simulink model "Droop"  (R2024b)
settings: Solver=VariableStepAuto  StartTime=0.0  StopTime=2  RelTol=1e-3
undefined symbols (not defined in the file): Ion, Lithium
libraries: spsSeriesRLCBranchLib x7, spsVoltageMeasurementLib x6, spsMosfetLib x4, spsCurrentMeasurementLib x3, spsBatteryLib x2, slpidlib x2, spsTriangleGeneratorLib x2, spsBreakerLib x1, spsPVArrayLib x1, spspowerguiLib x1
settings Model: Creator=ASUS  LastModifiedBy=ASUS

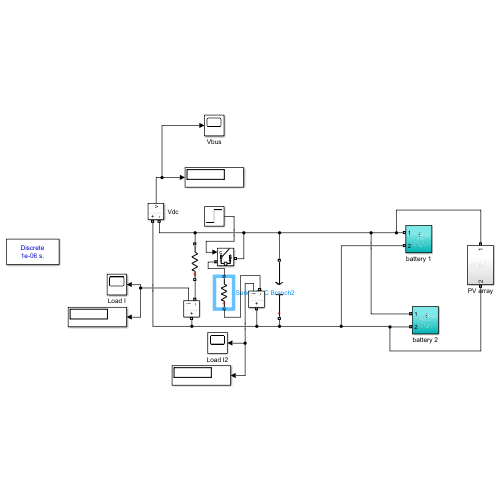
[thumbnail: Simulink's stored preview of the top-level diagram]
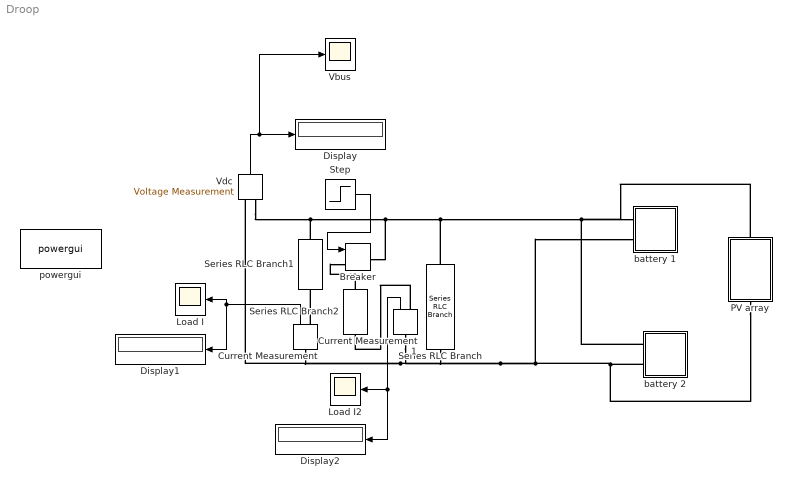
== system Droop ==
  Breaker : spsBreakerLib/Breaker  InitialState=0  SwitchingTimes="[1/60  5/60]"  External=on  BreakerResistance=0.01  SnubberResistance=1e6  SnubberCapacitance=inf  Measurements=None  MoreParameters=on  NoBreakLoop=off
  Current Measurement : spsCurrentMeasurementLib/Current Measurement  PhasorSimulation=off  OutputType=Complex  PSBequivalent=0
  Current Measurement1 : spsCurrentMeasurementLib/Current Measurement  PhasorSimulation=off  OutputType=Complex  PSBequivalent=0
  Display : Display
  Display1 : Display
  Display2 : Display
  Load I : Scope
  Load I2 : Scope
  PV array : Subsystem
      settings: PortSchema="{\"entries\":[{\"content\":{\"sides\":[{\"content\":{},\"type\":\"ConnectorPlacement.EquallySpacedRectSide\",\"uuid\":\"98c84815-b73a-4a68-a881-ea3acd4700a6\"},{\"content\":{\"side\":\"RIGHT\"},\"type\":\"ConnectorPlacement.EquallySpacedRectSide\",\"uuid\":\"a3c80d2d-1955-4a58-b743-6cecb5515e4f\"},{\"content\":{\"connectorIds\":[\"LConn1\"],\"side\":\"TOP\"},\"type\":\"ConnectorPlacement.EquallySpacedRectSide\",\"uuid\":\"fb99ad30-251c-48f2-b563-c26654c12262\"},{\"content\":{\"connectorIds\":[\"RConn1\"],\"side\":\"BOTTOM\"},\"type\":\"ConnectorPlacement.EquallySpacedRectSide\",\"uuid\":\"3c114dca-ead0-42e1-8f9f-90199643fe12\"}]},\"type\":\"ConnectorPlacement.EquallySpacedConnector\",\"uuid\":\"efc59635-4512-4ae2-8e03-d54fb94518f3\"}],\"packageUris\":[\"http://schema.mathworks.com/mf0/Connector/R2020b\"],\"version\":\"1.0\"}"
  Series RLC Branch : spsSeriesRLCBranchLib/Series RLC Branch  LConnTagsString=__new0  RConnTagsString=__new0  BranchType=C  Resistance=1  Inductance=1e-3  SetiL0=off  InitialCurrent=0  Capacitance=4700e-6  Setx0=off  InitialVoltage=0  Measurements=None
  Series RLC Branch1 : spsSeriesRLCBranchLib/Series RLC Branch  LConnTagsString=__new0  RConnTagsString=__new0  BranchType=R  Resistance=1  Inductance=1e-3  SetiL0=off  InitialCurrent=0  Capacitance=4700e-6  Setx0=off  InitialVoltage=0  Measurements=None
  Series RLC Branch2 : spsSeriesRLCBranchLib/Series RLC Branch  LConnTagsString=__new0  RConnTagsString=__new0  BranchType=R  Resistance=1  Inductance=1e-3  SetiL0=off  InitialCurrent=0  Capacitance=4700e-6  Setx0=off  InitialVoltage=0  Measurements=None
  Step : Step  Time=0.5  SampleTime=0
  Vbus : Scope
  Vdc : spsVoltageMeasurementLib/Voltage Measurement  PhasorSimulation=off  OutputType=Complex  PSBequivalent=0
  battery 1 : Subsystem
  battery 2 : Subsystem
  powergui : spspowerguiLib/powergui  Priority=1  SimulationMode=Discrete  SampleTime=1e-6  frequency=60  Iterations=50  frequencyindice=0  Pbase=100e6  ErrMax=1e-4  UnitsV=kV  UnitsW=MW  buscounter=0  FunctionMessages=off  echomessages=off  EnableUseOfTLC=off  CurrentSourceSwitches=off  DisableSnubberDevices=off  DisableRonSwitches=off  DisableVfSwitches=off  DisplayEquations=off  AutomaticDiscreteSolvers=off  SolverType=Tustin/Backward Euler (TBE)  Interpol=off  ExternalGateDelay=off  methode=off  Ts=100  x0status=blocks  SPID=on  SwTol=0  HookPort=off  NonlinearTolerance=1e-4  nMaxIteration=100  ContinueOnMaxIteration=off  RestoreLinks=warning  ResistiveCurrentMeasurement=off  Frange=[0:2:500]  Ylog=off  Xlog=on  ShowGrid=off  save=off  variable=ZData  structure=0  ZoomFFT=off  StartTime=0.0  cycles=1  DisplayStyle=1  fundamental=60  FreqAxis=off  MaxFrequency=1000  frequencyindicesteady=1  RmsSteady=1  display=off
  wires:
  Vdc/1 -> Vbus/1, Display/1
  Step/1 -> Breaker/1
  Current Measurement/1 -> Load I/1, Display1/1
  Current Measurement1/1 -> Display2/1, Load I2/1
  connections:
  battery 2/LConn2 -- battery 1/LConn2 -- Current Measurement/LConn1 -- Vdc/LConn1 -- Current Measurement1/LConn1 -- Series RLC Branch/LConn1 -- PV array/RConn1
  Vdc/LConn2 -- Series RLC Branch1/RConn1 -- Breaker/RConn1 -- Series RLC Branch/RConn1 -- PV array/LConn1 -- battery 1/LConn1 -- battery 2/LConn1
  Series RLC Branch2/RConn1 -- Breaker/LConn1
  Current Measurement/RConn1 -- Series RLC Branch1/LConn1
  Current Measurement1/RConn1 -- Series RLC Branch2/LConn1

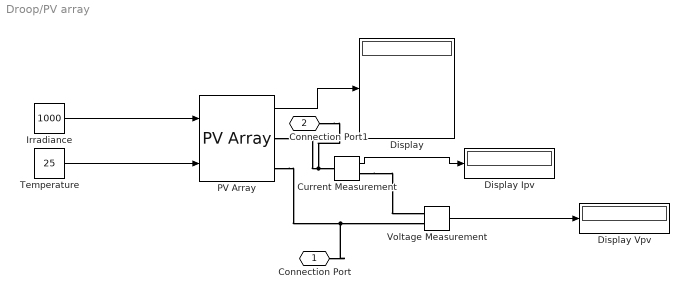
== system Droop/PV array ==
  Current Measurement : spsCurrentMeasurementLib/Current Measurement  PhasorSimulation=off  OutputType=Complex  PSBequivalent=0
  Display : Display
  Display Ipv : Display
  Display Vpv : Display
  Irradiance : Constant  Value=1000
  PV Array : spsPVArrayLib/PV Array  Npar=40  Nser=10  PlotType=array @ 1000 W/m2 & specified temperatures  S_vec="[ 1000  500  100 ]"  Temp_C_vec="[ 45 25  ]"  ModuleName=SunPower SPR-295E-WHT-D  PlotWhenSelected=off  Pm=295.39  Ncell=96  Voc=63.3  Isc=5.83  Vm=54.2  Im=5.45  beta_Voc_pc=-0.2727  alpha_Isc_pc=0.061732  beta_Voc=-0.17262  alpha_Isc=0.003599  IL=5.8532  I0=6.1666e-12  nI=0.93176  Rsh=315.2663  Rs=0.32243  RobustModel=off  RobustCellTemperature=313.3991  BAL=off  Tc=1e-6  Tfilter=5e-5
  Temperature : Constant  Value=25
  Voltage Measurement : spsVoltageMeasurementLib/Voltage Measurement  PhasorSimulation=off  OutputType=Complex  PSBequivalent=0
  Connection Port : PMIOPort  Side=Left
  Connection Port1 : PMIOPort  Port=2  Side=Right
  wires:
  Temperature/1 -> PV Array/2
  PV Array/1 -> Display/1
  Voltage Measurement/1 -> Display Vpv/1
  Irradiance/1 -> PV Array/1
  Current Measurement/1 -> Display Ipv/1
  connections:
  Current Measurement/RConn1 -- Voltage Measurement/LConn1
  PV Array/RConn2 -- Connection Port/RConn1 -- Voltage Measurement/LConn2
  PV Array/RConn1 -- Connection Port1/RConn1 -- Current Measurement/LConn1

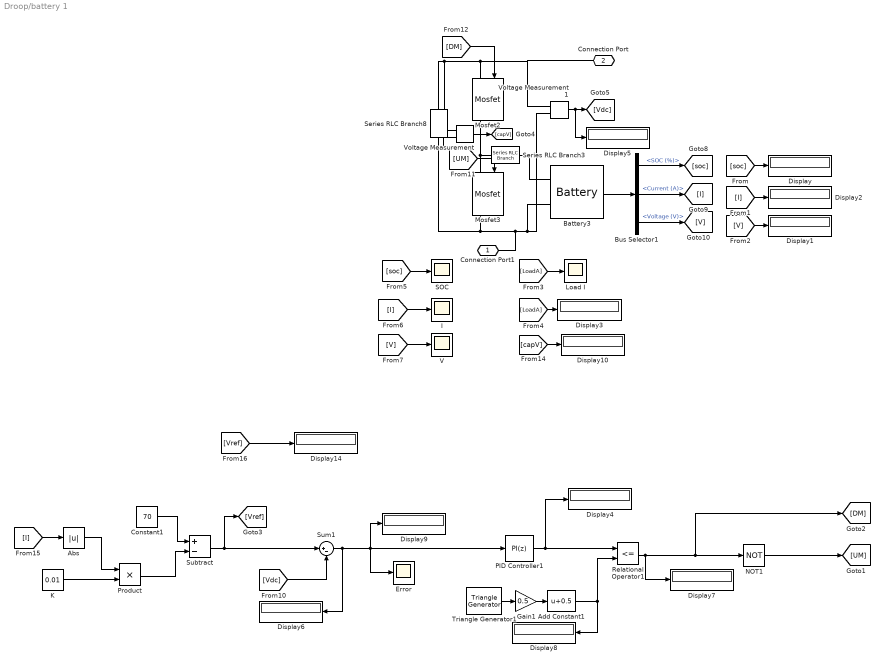
== system Droop/battery 1 ==
  Abs : Abs  SaturateOnIntegerOverflow=off
  Add Constant1 : Bias  Bias=0.5  SaturateOnIntegerOverflow=off
  Battery3 : spsBatteryLib/Battery  BatType=Lithium-Ion  NomV=50  NomQ=20  SOC=60  Batt_Tr=30  PresetModel=on  MaxQ=20  MinV=37.5  FullV=58.1994  Dis_rate=8.6957  R=0.025  Normal_OP=18.087  expZone="[54.0193     0.982609]"
  Bus Selector1 : BusSelector  OutputSignals=SOC (%),Current (A),Voltage (V)
  Constant1 : Constant  Value=70
  Display{,1..10,14} (12 alike) : Display
  Error : Scope
  Gain1 : Gain  Gain=0.5
  I : Scope
  K : Constant  Value=0.01
  Load I : Scope
  Mosfet2 : spsMosfetLib/Mosfet  Ron=0.1  Lon=0  Rd=0.01  Vfd=0  IC=0  Rs=1e6  Cs=inf  Measurements=on
  Mosfet3 : spsMosfetLib/Mosfet  Ron=0.1  Lon=0  Rd=0.01  Vfd=0  IC=0  Rs=1e6  Cs=inf  Measurements=on
  NOT1 : Logic  Operator=NOT  IconShape=distinctive  AllPortsSameDT=off  OutDataTypeStr=boolean
  PID Controller1 : slpidlib/PID Controller  Controller=PI  Form=Parallel  TimeDomain=Discrete-time  UseExternalTs=off  SampleTime=-1  IntegratorMethod=Forward Euler  FilterMethod=Forward Euler  ControllerParametersSource=internal  P=0.08  I=10  UseKiTs=off  D=0  UseExternalDerivativeSource=off  N=100  UseFilter=on  TunerSelectOption=Transfer Function Based (PID Tuner App)  ZeroCross=off  InitialConditionSource=internal  InitialConditionForIntegrator=0  InitialConditionForFilter=0  DifferentiatorICPrevScaledInput=0  ExternalReset=none  TrackingMode=off  Kt=1  LimitOutput=on  SatLimitsSource=internal  UpperSaturationLimit=1  LowerSaturationLimit=-1  LinearizeAsGain=on  AntiWindupMode=back-calculation  Kb=1  LimitIntegrator=off  UpperIntegratorSaturationLimit=inf  LowerIntegratorSaturationLimit=-inf  POutMin=[]  POutMax=[]  IOutMin=[]  IOutMax=[]  DOutMin=[]  DOutMax=[]  NOutMin=[]  NOutMax=[]  SumOutMin=[]  SumOutMax=[]  SaturationOutMin=[]  SaturationOutMax=[]  PParamMin=[]  PParamMax=[]  IParamMin=[]  IParamMax=[]  DParamMin=[]  DParamMax=[]  NParamMin=[]  NParamMax=[]  KbParamMin=[]  KbParamMax=[]  KtParamMin=[]  KtParamMax=[]  KbOutMin=[]  KbOutMax=[]  KtOutMin=[]  KtOutMax=[]  IntegratorOutMin=[]  IntegratorOutMax=[]  FilterOutMin=[]  FilterOutMax=[]  SumI1OutMin=[]  SumI1OutMax=[]  SumI2OutMin=[]  SumI2OutMax=[]  SumI3OutMin=[]  SumI3OutMax=[]  SumI4OutMin=[]  SumI4OutMax=[]  SumDOutMin=[]  SumDOutMax=[]  DifferentiatorOutMin=[]  DifferentiatorOutMax=[]  FilterDiffOutCoefMin=[]  FilterDiffOutCoefMax=[]  ReciprocalOutMin=[]  ReciprocalOutMax=[]  SumDenOutMin=[]  SumDenOutMax=[]  SumNumOutMin=[]  SumNumOutMax=[]  DivideOutMin=[]  DivideOutMax=[]  UdiffTsProdOutMin=[]  UdiffTsProdOutMax=[]  NTsProdOutMin=[]  NTsProdOutMax=[]  UintegralTsProdOutMin=[]  UintegralTsProdOutMax=[]  UngainTsProdOutMin=[]  UngainTsProdOutMax=[]  ClampingZeroOutDataTypeStr=Inherit: Inherit via back propagation  ClampingZeroOutMin=[]  ClampingZeroOutMax=[]  FilterDenConstantOutDataTypeStr=Inherit: Inherit via back propagation  FilterDenConstantOutMin=[]  FilterDenConstantOutMax=[]  PCopyOutDataTypeStr=Inherit: Inherit via back propagation  PCopyOutMin=[]  PCopyOutMax=[]  NCopyOutDataTypeStr=Inherit: Inherit via back propagation  NCopyOutMin=[]  NCopyOutMax=[]  IntegratorContinuousStateAttributes=''  IntegratorStateMustResolveToSignalObject=off  IntegratorRTWStateStorageClass=Auto  FilterContinuousStateAttributes=''  FilterStateMustResolveToSignalObject=off  FilterRTWStateStorageClass=Auto  ParallelPVariant=InternalParameters  IdealPVariant=Disabled  IVariant=InternalParameters  DVariant=Disabled  IntegratorVariant=Discrete  SatVariant=Enabled  AWVariant=BackCalculation  PCopyVariant=Disabled  TRVariant=Disabled  FdbkBlocksVariant=Forward  IdealPFdbkVariant=Disabled  SatFdbkVariant=Disabled  DerivativeFilterVariant=Disabled  NVariant=Disabled  NCopyVariant=Disabled_SignalSpec  FilterICVariant=Disabled  IntegratorICVariant=InternalICs  ExternalResetVariant=Disabled  TRSumVariant=Passthrough  SumFdbkVariant=Disabled  SumVariant=Sum_PI  TsampFilterVariant=InternalTs  TsampNgainVariant=Passthrough  TsampIntegralVariant=Disabled_SignalSpec  ExternalSaturationOutDataTypeStr=Inherit: Same as second input  DerivativeSourceVariant=Disabled  PreIntVariant=InternalPreInt
  Product : Product
  Relational Operator1 : RelationalOperator  Operator=<=  OutDataTypeStr=boolean  RndMeth=Simplest  InputSameDT=off
  SOC : Scope
  Series RLC Branch3 : spsSeriesRLCBranchLib/Series RLC Branch  LConnTagsString=__new0  RConnTagsString=__new0  BranchType=L  Resistance=1  Inductance=500e-6  SetiL0=off  InitialCurrent=0  Capacitance=1e-6  Setx0=off  InitialVoltage=0  Measurements=None
  Series RLC Branch8 : spsSeriesRLCBranchLib/Series RLC Branch  LConnTagsString=__new0  RConnTagsString=__new0  BranchType=RC  Resistance=1  Inductance=1e-3  SetiL0=off  InitialCurrent=0  Capacitance=1500e-6  Setx0=off  InitialVoltage=0  Measurements=None
  Subtract : Sum  Inputs=+-
  Sum1 : Sum  Inputs=|+-
  Triangle Generator1 : spsTriangleGeneratorLib/Triangle Generator  Freq=10000  Phase=0  Ts=1e-6
  V : Scope
  Voltage Measurement : spsVoltageMeasurementLib/Voltage Measurement  PhasorSimulation=off  OutputType=Complex  PSBequivalent=0
  Voltage Measurement1 : spsVoltageMeasurementLib/Voltage Measurement  PhasorSimulation=off  OutputType=Complex  PSBequivalent=0
  Connection Port1 : PMIOPort  Side=Left
  Connection Port : PMIOPort  Port=2  Side=Left
  wires:
  Voltage Measurement1/1 -> Display5/1, [Vdc]
  [UM] -> Mosfet3/1
  Add Constant1/1 -> Display8/1, Relational Operator1/2
  [V] -> Display1/1
  [capV] -> Display10/1
  [I] -> I/1
  Sum1/1 -> Display9/1, PID Controller1/1, Error/1, Display6/1
  Relational Operator1/1 -> [DM], NOT1/1, Display7/1
  Bus Selector1/1 -> [soc]  "<SOC (%)>"
  PID Controller1/1 -> Relational Operator1/1, Display4/1
  Gain1/1 -> Add Constant1/1
  [soc] -> SOC/1
  [I] -> Display2/1
  Battery3/1 -> Bus Selector1/1
  [DM] -> Mosfet2/1
  Bus Selector1/3 -> [V]  "<Voltage (V)>"
  [LoadA] -> Load I/1
  [V] -> V/1
  Voltage Measurement/1 -> [capV]
  [Vdc] -> Sum1/2
  [LoadA] -> Display3/1
  Triangle Generator1/1 -> Gain1/1
  Subtract/1 -> Sum1/1, [Vref]
  Bus Selector1/2 -> [I]  "<Current (A)>"
  [soc] -> Display/1
  [I] -> Abs/1
  Abs/1 -> Product/1
  K/1 -> Product/2
  Product/1 -> Subtract/2
  Constant1/1 -> Subtract/1
  NOT1/1 -> [UM]
  [Vref] -> Display14/1
  connections:
  Battery3/LConn1 -- Series RLC Branch3/LConn1
  Series RLC Branch8/LConn1 -- Voltage Measurement1/LConn1 -- Connection Port/RConn1 -- Mosfet2/LConn1 -- Voltage Measurement/LConn1
  Battery3/LConn2 -- Connection Port1/RConn1 -- Series RLC Branch8/RConn1 -- Voltage Measurement/LConn2 -- Mosfet3/RConn1 -- Voltage Measurement1/LConn2
  Mosfet2/RConn1 -- Series RLC Branch3/RConn1 -- Mosfet3/LConn1

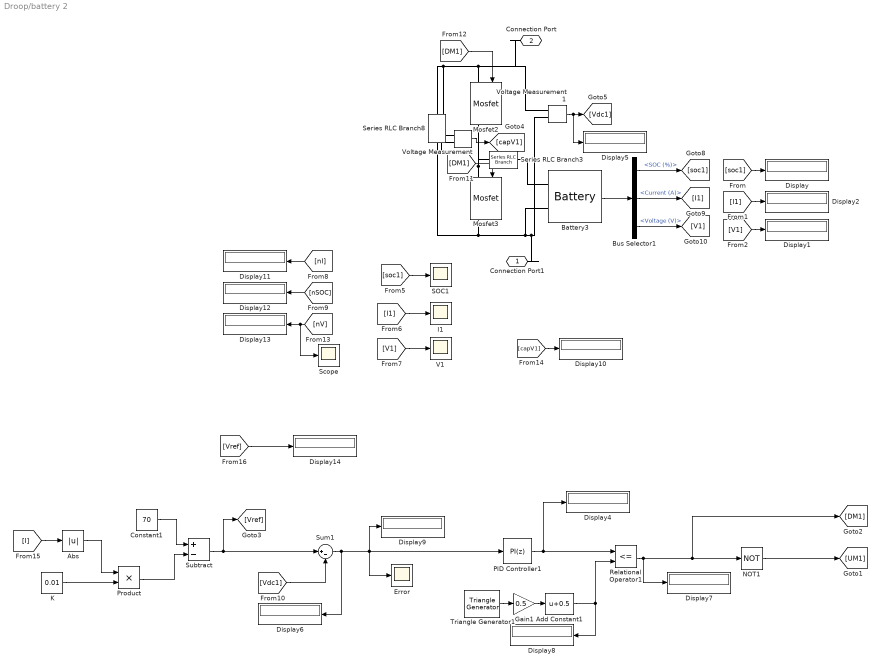
== system Droop/battery 2 ==
  Abs : Abs  SaturateOnIntegerOverflow=off
  Add Constant1 : Bias  Bias=0.5  SaturateOnIntegerOverflow=off
  Battery3 : spsBatteryLib/Battery  BatType=Lithium-Ion  NomV=50  NomQ=20  SOC=60  Batt_Tr=30  PresetModel=on  MaxQ=20  MinV=37.5  FullV=58.1994  Dis_rate=8.6957  R=0.025  Normal_OP=18.087  expZone="[54.0193     0.982609]"
  Bus Selector1 : BusSelector  OutputSignals=SOC (%),Current (A),Voltage (V)
  Constant1 : Constant  Value=70
  Display{,1..2,4..14} (14 alike) : Display
  Error : Scope
  Gain1 : Gain  Gain=0.5
  I1 : Scope
  K : Constant  Value=0.01
  Mosfet2 : spsMosfetLib/Mosfet  Ron=0.1  Lon=0  Rd=0.01  Vfd=0  IC=0  Rs=1e6  Cs=inf  Measurements=on
  Mosfet3 : spsMosfetLib/Mosfet  Ron=0.1  Lon=0  Rd=0.01  Vfd=0  IC=0  Rs=1e6  Cs=inf  Measurements=on
  NOT1 : Logic  Operator=NOT  IconShape=distinctive  AllPortsSameDT=off  OutDataTypeStr=boolean
  PID Controller1 : slpidlib/PID Controller  Controller=PI  Form=Parallel  TimeDomain=Discrete-time  UseExternalTs=off  SampleTime=-1  IntegratorMethod=Forward Euler  FilterMethod=Forward Euler  ControllerParametersSource=internal  P=0.08  I=10  UseKiTs=off  D=0  UseExternalDerivativeSource=off  N=100  UseFilter=on  TunerSelectOption=Transfer Function Based (PID Tuner App)  ZeroCross=off  InitialConditionSource=internal  InitialConditionForIntegrator=0  InitialConditionForFilter=0  DifferentiatorICPrevScaledInput=0  ExternalReset=none  TrackingMode=off  Kt=1  LimitOutput=on  SatLimitsSource=internal  UpperSaturationLimit=1  LowerSaturationLimit=-1  LinearizeAsGain=on  AntiWindupMode=back-calculation  Kb=1  LimitIntegrator=off  UpperIntegratorSaturationLimit=inf  LowerIntegratorSaturationLimit=-inf  POutMin=[]  POutMax=[]  IOutMin=[]  IOutMax=[]  DOutMin=[]  DOutMax=[]  NOutMin=[]  NOutMax=[]  SumOutMin=[]  SumOutMax=[]  SaturationOutMin=[]  SaturationOutMax=[]  PParamMin=[]  PParamMax=[]  IParamMin=[]  IParamMax=[]  DParamMin=[]  DParamMax=[]  NParamMin=[]  NParamMax=[]  KbParamMin=[]  KbParamMax=[]  KtParamMin=[]  KtParamMax=[]  KbOutMin=[]  KbOutMax=[]  KtOutMin=[]  KtOutMax=[]  IntegratorOutMin=[]  IntegratorOutMax=[]  FilterOutMin=[]  FilterOutMax=[]  SumI1OutMin=[]  SumI1OutMax=[]  SumI2OutMin=[]  SumI2OutMax=[]  SumI3OutMin=[]  SumI3OutMax=[]  SumI4OutMin=[]  SumI4OutMax=[]  SumDOutMin=[]  SumDOutMax=[]  DifferentiatorOutMin=[]  DifferentiatorOutMax=[]  FilterDiffOutCoefMin=[]  FilterDiffOutCoefMax=[]  ReciprocalOutMin=[]  ReciprocalOutMax=[]  SumDenOutMin=[]  SumDenOutMax=[]  SumNumOutMin=[]  SumNumOutMax=[]  DivideOutMin=[]  DivideOutMax=[]  UdiffTsProdOutMin=[]  UdiffTsProdOutMax=[]  NTsProdOutMin=[]  NTsProdOutMax=[]  UintegralTsProdOutMin=[]  UintegralTsProdOutMax=[]  UngainTsProdOutMin=[]  UngainTsProdOutMax=[]  ClampingZeroOutDataTypeStr=Inherit: Inherit via back propagation  ClampingZeroOutMin=[]  ClampingZeroOutMax=[]  FilterDenConstantOutDataTypeStr=Inherit: Inherit via back propagation  FilterDenConstantOutMin=[]  FilterDenConstantOutMax=[]  PCopyOutDataTypeStr=Inherit: Inherit via back propagation  PCopyOutMin=[]  PCopyOutMax=[]  NCopyOutDataTypeStr=Inherit: Inherit via back propagation  NCopyOutMin=[]  NCopyOutMax=[]  IntegratorContinuousStateAttributes=''  IntegratorStateMustResolveToSignalObject=off  IntegratorRTWStateStorageClass=Auto  FilterContinuousStateAttributes=''  FilterStateMustResolveToSignalObject=off  FilterRTWStateStorageClass=Auto  ParallelPVariant=InternalParameters  IdealPVariant=Disabled  IVariant=InternalParameters  DVariant=Disabled  IntegratorVariant=Discrete  SatVariant=Enabled  AWVariant=BackCalculation  PCopyVariant=Disabled  TRVariant=Disabled  FdbkBlocksVariant=Forward  IdealPFdbkVariant=Disabled  SatFdbkVariant=Disabled  DerivativeFilterVariant=Disabled  NVariant=Disabled  NCopyVariant=Disabled_SignalSpec  FilterICVariant=Disabled  IntegratorICVariant=InternalICs  ExternalResetVariant=Disabled  TRSumVariant=Passthrough  SumFdbkVariant=Disabled  SumVariant=Sum_PI  TsampFilterVariant=InternalTs  TsampNgainVariant=Passthrough  TsampIntegralVariant=Disabled_SignalSpec  ExternalSaturationOutDataTypeStr=Inherit: Same as second input  DerivativeSourceVariant=Disabled  PreIntVariant=InternalPreInt
  Product : Product
  Relational Operator1 : RelationalOperator  Operator=<=  OutDataTypeStr=boolean  RndMeth=Simplest  InputSameDT=off
  SOC1 : Scope
  Scope : Scope
  Series RLC Branch3 : spsSeriesRLCBranchLib/Series RLC Branch  LConnTagsString=__new0  RConnTagsString=__new0  BranchType=L  Resistance=1  Inductance=500e-6  SetiL0=off  InitialCurrent=0  Capacitance=1e-6  Setx0=off  InitialVoltage=0  Measurements=None
  Series RLC Branch8 : spsSeriesRLCBranchLib/Series RLC Branch  LConnTagsString=__new0  RConnTagsString=__new0  BranchType=RC  Resistance=1  Inductance=1e-3  SetiL0=off  InitialCurrent=0  Capacitance=1500e-6  Setx0=off  InitialVoltage=0  Measurements=None
  Subtract : Sum  Inputs=+-
  Sum1 : Sum  Inputs=|+-
  Triangle Generator1 : spsTriangleGeneratorLib/Triangle Generator  Freq=10000  Phase=0  Ts=1e-6
  V1 : Scope
  Voltage Measurement : spsVoltageMeasurementLib/Voltage Measurement  PhasorSimulation=off  OutputType=Complex  PSBequivalent=0
  Voltage Measurement1 : spsVoltageMeasurementLib/Voltage Measurement  PhasorSimulation=off  OutputType=Complex  PSBequivalent=0
  Connection Port1 : PMIOPort  Side=Left
  Connection Port : PMIOPort  Port=2  Side=Left
  wires:
  [Vref] -> Display14/1
  NOT1/1 -> [UM1]
  Constant1/1 -> Subtract/1
  Product/1 -> Subtract/2
  K/1 -> Product/2
  Abs/1 -> Product/1
  [I] -> Abs/1
  [soc1] -> Display/1
  Bus Selector1/2 -> [I1]  "<Current (A)>"
  Subtract/1 -> [Vref], Sum1/1
  Triangle Generator1/1 -> Gain1/1
  [Vdc1] -> Sum1/2
  Voltage Measurement/1 -> [capV1]
  [nSOC] -> Display12/1
  [V1] -> V1/1
  [nI] -> Display11/1
  Bus Selector1/3 -> [V1]  "<Voltage (V)>"
  [DM1] -> Mosfet2/1
  Battery3/1 -> Bus Selector1/1
  [I1] -> Display2/1
  [soc1] -> SOC1/1
  Gain1/1 -> Add Constant1/1
  [nV] -> Display13/1, Scope/1
  PID Controller1/1 -> Display4/1, Relational Operator1/1
  Bus Selector1/1 -> [soc1]  "<SOC (%)>"
  Relational Operator1/1 -> Display7/1, NOT1/1, [DM1]
  Sum1/1 -> Display6/1, Error/1, PID Controller1/1, Display9/1
  [I1] -> I1/1
  [capV1] -> Display10/1
  [V1] -> Display1/1
  Add Constant1/1 -> Relational Operator1/2, Display8/1
  [DM1] -> Mosfet3/1
  Voltage Measurement1/1 -> [Vdc1], Display5/1
  connections:
  Mosfet3/LConn1 -- Series RLC Branch3/RConn1 -- Mosfet2/RConn1
  Voltage Measurement1/LConn2 -- Connection Port1/RConn1 -- Mosfet3/RConn1 -- Voltage Measurement/LConn2 -- Series RLC Branch8/RConn1 -- Battery3/LConn2
  Voltage Measurement/LConn1 -- Connection Port/RConn1 -- Voltage Measurement1/LConn1 -- Mosfet2/LConn1 -- Series RLC Branch8/LConn1
  Battery3/LConn1 -- Series RLC Branch3/LConn1
